simulink model "Ro_contributions"  (R2021a)
settings: Solver=VariableStepAuto  StartTime=0.0  StopTime=1  RelTol=1e-3
undefined symbols (not defined in the file or in its folder): newDymolaGui
settings Model: Creator=jason  LastModifiedBy=jason

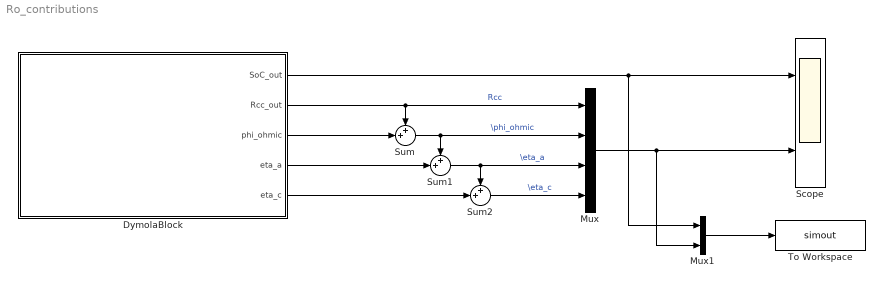
== system Ro_contributions ==
  DymolaBlock : Subsystem  Tag=21-Aug-2022 21:54:25#9058
      mask help:
      | Dymola block.
      | A dymola block allows acausal physical modeling.
      | See Dymola manual for usage.
      settings: CopyFcn=newDymolaGui('21-Aug-2022 21:54:25#9058','Copy');  DeleteFcn=if exist('newDymolaGui') newDymolaGui('Ro_contributions/DymolaBlock','Delete'); end;  NameChangeFcn=newDymolaGui('21-Aug-2022 21:54:25#9058','Copy');  OpenFcn=newDymolaGui('Ro_contributions/DymolaBlock','Init');
      mask Display: image(imread('Dymola.bmp'),[.2,.2,.6,.6])
  Mux : Mux
  Mux1 : Mux  Inputs=2
  Scope : Scope  NumInputPorts=2
  Sum : Sum  Inputs=++|
  Sum1 : Sum  Inputs=++|
  Sum2 : Sum  Inputs=++|
  To Workspace : ToWorkspace  VariableName=simout  SaveFormat=Timeseries  SampleTime=-1
  wires:
  DymolaBlock/5(eta_c) -> Sum2/2
  DymolaBlock/4(eta_a) -> Sum1/2
  Sum1/1 -> Mux/3, Sum2/1  "\\eta_a"
  Sum/1 -> Sum1/1, Mux/2  "\\phi_ohmic"
  DymolaBlock/3(phi_ohmic) -> Sum/2
  DymolaBlock/2(Rcc_out) -> Sum/1, Mux/1  "Rcc"
  DymolaBlock/1(SoC_out) -> Mux1/1, Scope/1
  Sum2/1 -> Mux/4  "\\eta_c"
  Mux/1 -> Mux1/2, Scope/2
  Mux1/1 -> To Workspace/1

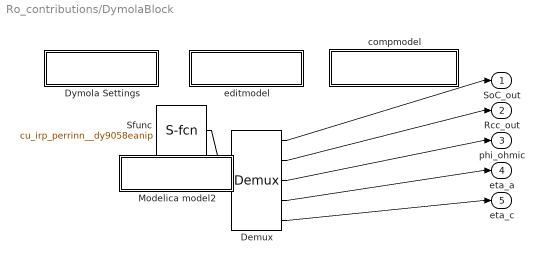
== system Ro_contributions/DymolaBlock ==
  Demux : Demux  Outputs=[1;1;1;1;1]
  Dymola Settings : Subsystem  mask{ModelName=CU_IRP_perrinn_battery.Test_Bench.Sketch, MoFileName=C:/Users/jason/OneDrive - The Hong Kong Polytechnic University/Cranfield Studies/4 Course Projects/IRP Battery/dymola_git/CU_IRP_perrinn_battery/Test_Bench/Sketch.mo, dSpace=, BusConnector=[], ResultFile=[], ResultFileOnline=[], ResultDt=[], Libs=:, bigobj=[], ImportFolder=[], guimode=[], ModelName2=[], forRuntime=[], MEXLoad=[], omitDescription=[], ResultName=cu_irp_perrinn__dy9058eanip}
      mask prompts: ModelName "Name of Dymola model"; MoFileName "File Name (including .mo)"; ResultFile "Create Result"; ResultFileOnline "Load result"; ResultDt "Result min dt"; Libs "Used Libraries"; bigobj "Compiler flag /bigobj"; ImportFolder "Import folder"; guimode "GUI mode flag"; ModelName2 "Model name for import mode"; forRuntime "Runtime export"; MEXLoad "Compiled S-function"; omitDescription "Omit description strings"; ResultName "Name of result file"
      mask Display: disp('Dymola Settings');
  Modelica model2 : Subsystem
      mask Display: disp('Change parameters');
  Sfunc : S-Function  Tag=9058eanip  FunctionName=cu_irp_perrinn__dy9058eanip  Parameters=[Temp_k;radius_c_k;ro_multiSum_significantDi3;ro_multiSum_k;ro_sigma_e1_T_square_sign5;ro_sigma_e1_K00_k;ro_sigma_e1_multiSum_sign7;ro_sigma_e1_multiSum_k;ro_sigma_e1_K01_k;ro_sigma_e1_K02_k;ro_sigma_e1_K11_k;ro_sigma_e1_K12_k;ro_sigma_e1_K21_k;ro_sigma_e1_K20_k;ro_sigma_e1_K10_k;ro_sigma_e1_add3_1_k1;ro_sigma_e1_add3_1_k2;ro_sigma_e1_add3_1_k3;ro_sigma_e1_add_k1;ro_sigma_e1_add_k2;ro_sigma_e1_Gain_k;ro_a_c_gain_k;ro_a_a_gain_k;ro_multiProduct_significa24;ro_multiProduct1_signific25;Lc_k;Ls_k;La_k;Rcc_k;A_k;Rbar_k;F_k;epsilon_c_k;epsilon_a_k;radius_a_k;Ce_0_k;SoC_height;SoC_duration;SoC_offset;SoC_startTime;c_max_c_k;c_max_a_k;kc_k;ka_k;theta_0_c_k;theta_0_a_k;theta_100_c_k;theta_100_a_k;Ea_i_o_c_k;Ea_i_o_a_k;Tref_k],[]  PortCounts=[0;1]  SFunctionDeploymentMode=off  EnableBusSupport=off  mask{Temp_k=298.15, radius_c_k=4e-06, ro_multiSum_significantDi3=3, ro_multiSum_k=[1; 1; 1; 1], ro_sigma_e1_T_square_sign5=3, ro_sigma_e1_K00_k=-10.5, ro_sigma_e1_multiSum_sign7=3, ro_sigma_e1_multiSum_k=[1; 1; 1; 1; 1], ro_sigma_e1_K01_k=0.074, ro_sigma_e1_K02_k=-6.96e-05, ro_sigma_e1_K11_k=-0.0178, ro_sigma_e1_K12_k=2.8e-05, ro_sigma_e1_K21_k=-0.000886, ro_sigma_e1_K20_k=0.494, ro_sigma_e1_K10_k=0.668, ro_sigma_e1_add3_1_k1=1, ro_sigma_e1_add3_1_k2=1, ro_sigma_e1_add3_1_k3=1, ro_sigma_e1_add_k1=1, ro_sigma_e1_add_k2=1, ro_sigma_e1_Gain_k=0.1, ro_a_c_gain_k=3, ro_a_a_gain_k=3, ro_multiProduct_significa24=3, ro_multiProduct1_signific25=3, Lc_k=7.5e-05, Ls_k=2e-05, La_k=7e-05, Rcc_k=0.0004, A_k=2, Rbar_k=8.314, F_k=96500, epsilon_c_k=0.546, epsilon_a_k=0.51, radius_a_k=3e-06, Ce_0_k=1000, SoC_height=1, SoC_duration=1, SoC_offset=0, SoC_startTime=0, c_max_c_k=43000, c_max_a_k=31300, kc_k=3e-11, ka_k=9e-11, theta_0_c_k=0.9903, theta_0_a_k=0.0621, theta_100_c_k=0.4384, theta_100_a_k=0.9373, Ea_i_o_c_k=55200, Ea_i_o_a_k=6280, Tref_k=293.15}
      mask prompts: Temp_k "Temp.k"; radius_c_k "radius_c.k"; ro_multiSum_significantDi3 "ro.multiSum.significantDigits"; ro_multiSum_k "ro.multiSum.k"; ro_sigma_e1_T_square_sign5 "ro.sigma_e1.T_square.significantDigits"; ro_sigma_e1_K00_k "ro.sigma_e1.K00.k"; ro_sigma_e1_multiSum_sign7 "ro.sigma_e1.multiSum.significantDigits"; ro_sigma_e1_multiSum_k "ro.sigma_e1.multiSum.k"; ro_sigma_e1_K01_k "ro.sigma_e1.K01.k"; ro_sigma_e1_K02_k "ro.sigma_e1.K02.k"; ro_sigma_e1_K11_k "ro.sigma_e1.K11.k"; ro_sigma_e1_K12_k "ro.sigma_e1.K12.k"; ro_sigma_e1_K21_k "ro.sigma_e1.K21.k"; ro_sigma_e1_K20_k "ro.sigma_e1.K20.k"; ro_sigma_e1_K10_k "ro.sigma_e1.K10.k"; ro_sigma_e1_add3_1_k1 "ro.sigma_e1.add3_1.k1"; ro_sigma_e1_add3_1_k2 "ro.sigma_e1.add3_1.k2"; ro_sigma_e1_add3_1_k3 "ro.sigma_e1.add3_1.k3"; ro_sigma_e1_add_k1 "ro.sigma_e1.add.k1"; ro_sigma_e1_add_k2 "ro.sigma_e1.add.k2"; ro_sigma_e1_Gain_k "ro.sigma_e1.Gain.k"; ro_a_c_gain_k "ro.a_c.gain.k"; ro_a_a_gain_k "ro.a_a.gain.k"; ro_multiProduct_significa24 "ro.multiProduct.significantDigits"; ro_multiProduct1_signific25 "ro.multiProduct1.significantDigits"; Lc_k "Lc.k"; Ls_k "Ls.k"; La_k "La.k"; Rcc_k "Rcc.k"; A_k "A.k"; Rbar_k "Rbar.k"; F_k "F.k"; epsilon_c_k "epsilon_c.k"; epsilon_a_k "epsilon_a.k"; radius_a_k "radius_a.k"; Ce_0_k "Ce_0.k"; SoC_height "SoC.height"; SoC_duration "SoC.duration"; SoC_offset "SoC.offset"; SoC_startTime "SoC.startTime"; c_max_c_k "c_max_c.k"; c_max_a_k "c_max_a.k"; kc_k "kc.k"; ka_k "ka.k"; theta_0_c_k "theta_0_c.k"; theta_0_a_k "theta_0_a.k"; theta_100_c_k "theta_100_c.k"; theta_100_a_k "theta_100_a.k"; Ea_i_o_c_k "Ea_i_o_c.k"; Ea_i_o_a_k "Ea_i_o_a.k"; Tref_k "Tref.k"
      mask Display: image(imread('Dymola.bmp'))
  compmodel : Subsystem  InitFcn=newDymolaGui('Ro_contributions/DymolaBlock','Verify');
      settings: OpenFcn=compileModelica('Ro_contributions/DymolaBlock');
      mask Display: disp('Compile Modelica model');
  editmodel : Subsystem
      settings: OpenFcn=editModelica('Ro_contributions/DymolaBlock');
      mask Display: disp('Edit Modelica model');
  SoC_out : Outport
  Rcc_out : Outport  Port=2
  phi_ohmic : Outport  Port=3
  eta_a : Outport  Port=4
  eta_c : Outport  Port=5
  wires:
  Sfunc/1 -> Demux/1
  Demux/1 -> SoC_out/1
  Demux/2 -> Rcc_out/1
  Demux/3 -> phi_ohmic/1
  Demux/4 -> eta_a/1
  Demux/5 -> eta_c/1

== system Ro_contributions/DymolaBlock/Dymola Settings ==

== system Ro_contributions/DymolaBlock/Modelica model2 ==

== system Ro_contributions/DymolaBlock/compmodel ==

== system Ro_contributions/DymolaBlock/editmodel ==
